simulink library "lego_nxt_lib"  (Simulink 7.5)
settings: Solver=ode45  SolverMode=SingleTasking  StartTime=0.0  StopTime=10.0  RelTol=1e-3
undefined symbols (not defined in the file or in its folder): Copy_of_lego_nxt_lib, PWM
libraries: simulink x1
settings Model: Creator=cmcart01  LastModifiedBy=jpeytonj

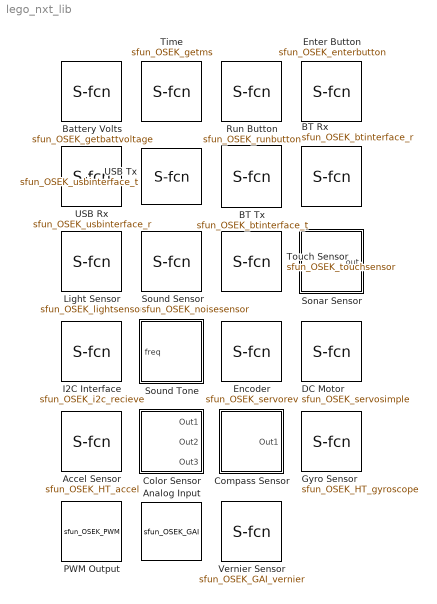
== system lego_nxt_lib ==
  Accel Sensor : S-Function  FunctionName=sfun_OSEK_HT_accel  Parameters=port, st  EnableBusSupport=off  mask(HiTechnic Acceleration Sensor){port=Port 1, st=-1}
      mask prompts: st "Sample time (-1 for inherited):"
      mask help: Outputs acceleration data in three axes (x, y and z) [uint16] representing forward, lateral and vertical directions respectively. The outputs are given in the range 0 to 1023 with a scale factor of ~200 units per g.
      mask init:
      | port_disp(gcb)
      mask Help:
      | The <b>Acceleration Sensor</b> block is an interface for the HiTechnic
      | Accelerometer for the Lego NXT brick.  This sensor can detect values in
      | three axes: x (or pitch), y (or roll) and z.  Pitch represents the angle
      | above or below the horizontal, while roll represents the angle left or
      | right of perfectly vertical.  The z-axis represents lean forward or
      | backward.
      mask StyleString: popup(Port 1|Port 2|Port 3|Port 4),edit
      mask Display:
      | image(imread('ht.jpg'))
      | port_label('output', 1, 'x')
      | port_label('output', 2, 'y')
      | port_label('output', 3, 'z')
      | text(0.1,0.15,'1')
  Analog Input : S-Function  FunctionName=sfun_OSEK_GAI  Parameters=port,gain,intercept,sign,st  EnableBusSupport=off  mask(Generic Analog Input for Mindstorms){port=Port 3, units=Raw ADC count [uint16]; range [0 1023], gain=1, intercept=0, sign=0, st=-1}
      mask prompts: units "Units of Measure:"; sign "Signed output"; st "Sample time (-1 for inherited)"
      mask help:
      | y = ((ADC count)*Gain + Intercept) / 100000.
      | The linear gain and intercept calibration constants are automatically defined for any specified sensor, but may be entered manually for the 'User Defined' measurement option.
      mask init:
      | port_disp(gcb)
      | sens_disp(gcb)
      mask Help:
      | The <b>Generic Analog Input</b> block is an interface for most of the
      | Mindstorms sensors for the Lego NXT brick.
      | 
      | The calibrated output, y, uses linear scaling according to: y = ((ADC count)*Gain + Intercept) / 100000
      | 
      | The relevant values are set automatically according to Mindstorms' documentation which may be found <a href="http://lejos-osek.sourceforge.net/ecrobot_c_api_frame.htm">here</a>
      mask StyleString: popup(Port 1|Port 2|Port 3|Port 4),popup(User defined|Raw ADC count [uint16]; range [0 1023]|Voltage [int16]; range [0 5]V|Light Intensity [uint16]; range [0 1023]|Sound Intensity [uint16]; range [0 1023]),edit,edit,edit,edit
      mask CallbackString:
      | |set_param(gcb,'MaskEnables',{'on','on','off','off','off','on'});
      | temp = get_param(gcb, 'MaskValues');
      | switch get_param(gcb,'units')
      | %NOTE: These are in no particular order as of now
      |     case 'Raw ADC count [uint16]; range [0 1023]'
      |         temp{3} = '1';
      |         temp{4} = '0';
      |         temp{5} = '0';
      |     case 'Voltage [int16]; range [0 5]V'
      |         temp{3} = '.00489';
      |         temp{4} = '0';
      |         temp{5} = '1';
      |     case 'Light Intensity [uint16]; range [0 1023]'
      |         temp{3} = '-1';
      |         temp{4} = '1023';
      |         temp{5} = '0';
      |     case 'Sound Intensity [uint16]; range [0 1023]'
      |         temp{3} = '-1';
      |         temp{4} = '1023';
      |         temp{5} = '0';
      |     case 'User Defined'
      |         set_param(gcb,'MaskEnables',{'on','on','on','on','off','on'});
      |     otherwise
      |         temp{3} = '1';
      |         temp{4} = '0';
      |         temp{5} = '0';
      | end;
      | 
      | set_param(gcb, 'MaskValues', temp);||||
      mask Display:
      | text(0.1,0.15,'3');
      | disp('Raw ADC Count');
  BT Rx : S-Function  AncestorBlock=lego_nxt_lib/USB Rx  FunctionName=sfun_OSEK_btinterface_r  Parameters=init_y0, st  EnableBusSupport=off  mask(Bluetooth Rx Interface    ){init_y0=zeros(32,1,'uint8'), mos=Slave, ip=0, st=-1}
      mask prompts: init_y0 "Initial Output [32x1]uint8:"; mos "Master or Slave"; ip "Slave Device Address:"; st "Sample Time (-1 for inherited):"
      mask help: Receives uint8 vector data via Bluetooth connection. The 'size' secondary output returns the number of bytes received in the last transmission [uint8]. Do not send more than 32 bytes in one timestep; doing so may cause unexpected functionality.
      mask Help:
      | The <b>BT Rx Interface</b> block allows the Lego NXT brick to easily recieve
      | data from an outside machine via Bluetooth. This block should be used only once
      | in a model. It can only receive byte vectors (uint8 vectors). The size
      | output gives the size of the vector received from the current connection.
      | Max vector size for recieve is 32 bytes
      mask StyleString: edit,popup(Master|Slave),edit,edit
      mask CallbackString:
      | |switch (get_param(gcb,'mos'))
      |     case 'Slave'
      |     set_param(gcb,'MaskEnables',{'on','on','off','on'});
      |     set_param(gcb,'MaskVisibilities',{'on','on','off','on'});
      |     case 'Master'
      |     set_param(gcb,'MaskEnables',{'on','on','on','on'});
      |     set_param(gcb,'MaskVisibilities',{'on','on','on','on'});
      | end
      | 
      | ||
      mask Display:
      | image(imread('bt.jpg'), [.2,.1,.6,.8])
      | port_label('output', 1, 'Rx')
      | port_label('output', 2, 'size')
  BT Tx : S-Function  FunctionName=sfun_OSEK_btinterface_t  EnableBusSupport=off  mask(Bluetooth Tx Interface){mos=Slave, ip=0}
      mask prompts: mos "Master or Slave:"; ip "Slave Device Address:"
      mask help: Transmits uint8 vector data via Bluetooth connection. Do not send more than 64 bytes in one timestep; doing so may cause unexpected functionality.
      mask Help:
      | The <b>BT Tx Interface</b> block allows the Lego NXT brick to easily transmit
      | data to an outside machine via Bluetooth. This block should be used only once
      | in a model. It can only transmit byte vectors (uint8 vectors). Max vector
      | size for transmit is 32 bytes.
      mask StyleString: popup(Master|Slave),edit
      mask CallbackString:
      | switch (get_param(gcb,'mos'))
      |     case 'Slave'
      |     set_param(gcb,'MaskEnables',{'on','off'});
      |     set_param(gcb,'MaskVisibilities',{'on','off'});
      |     case 'Master'
      |     set_param(gcb,'MaskEnables',{'on','on'});
      |     set_param(gcb,'MaskVisibilities',{'on','on'});
      | end
      | |
      mask Display:
      | image(imread('bt.jpg'), [.2,.1,.6,.8])
      | port_label('input', 1, 'Tx')
  Battery Volts : S-Function  FunctionName=sfun_OSEK_getbattvoltage  Parameters=st  EnableBusSupport=off  mask(Battery Voltage){st=-1}
      mask prompts: st "Sample time (-1 for inherited):"
      mask help: Outputs current source voltage of battery in mV [uint16].
      mask Help:
      | The <b>Battery Voltage</b> block will output the current source voltage at
      | the battery in mV.  For example, an output of 9000 represents 9.0 V.
      | Maximum value is ideally 9000.
      mask Display: image(imread('volt.jpg'),[.2,.2,.6,.6],'on')
  Color Sensor : Subsystem  mask(HiTechnic Color Sensor V2){port=Port 1, st=-1}
      mask prompts: st "Sample time (-1 for inherited)"
      mask help: Outputs red, green, and blue color saturation values [int16]. Values of each element range from 0-255.
      mask init:
      | port_disp(gcb)
      mask Help:
      | The <b>Color Sensor </b> block reads raw data from a color sensor and
      | extracts the RGB value of a color from that data. The values of each hue are
      | ranged between 0 and 255, as per normal RGB format. This block does not
      | implement the "color number" format supported by the color sensor.
      mask StyleString: popup(Port 1|Port 2|Port 3|Port 4),edit
      mask Display:
      | image(imread('htc.jpg'))
      | text(0.1,0.15,'1')
      | port_label('output', 1, 'r')
      | port_label('output', 2, 'g')
      | port_label('output', 3, 'b')
  Compass Sensor : Subsystem  mask(HiTechnic Compass Sensor   ){port=Port 1, st=-1}
      mask prompts: st "Sample time (-1 for inherited):"
      mask help: Outputs directional data [S16] relative to the closest magnetic source (or magnetic north, by default) in the range of [1,179].
      mask init:
      | port_disp(gcb)
      mask Help:
      | The <b>Compass Sensor</b> block is an interface for HiTechnic's Compass
      | for the Lego NXT brick.  This sensor determines the direction your robot is
      | pointing, which is referred to as the compass heading. The compass outputs
      | a range of values from 1-179, which equals the compass heading divided
      | by 2. The compass may be subject to interference from other magnetic
      | devices, including the brick and motors of the robot itself, so it is
      | important to mount the sensor at least 6 inches away from these objects.
      mask StyleString: popup(Port 1|Port 2|Port 3|Port 4),edit
      mask Display:
      | image(imread('ht.jpg'))
      | text(0.1,0.15,'1')
  DC Motor : S-Function  FunctionName=sfun_OSEK_servosimple  Parameters=port,brake  EnableBusSupport=off  mask(Servo Motor (Simple)){port=Port A, brake=Coast}
      mask prompts: brake "When power=0..."
      mask help: Sets the applied motor voltage [int8] as a percentage (in the range -100..100) of battery voltage. Applying a negative voltage will cause the motor to turn in the reverse direction. Note that motor speed depends not only on applied voltage, but also on motor load.
      mask init:
      | port_disp(gcb)
      mask Help:
      | The <b>DC Motor</b> block is a simplified interface for setting
      | Servo Motor speed.
      mask StyleString: popup(Port A|Port B|Port C),popup(Coast|Brake)
      mask Display:
      | image(imread('servo.jpg'))
      | text(0.1,0.15,'A')
  Encoder : S-Function  FunctionName=sfun_OSEK_servorev  Parameters=port, st  EnableBusSupport=off  mask(Encoder){port=Port A, st=-1}
      mask prompts: st "Sample time (-1 for inherited):"
      mask help: Counts encoder pulses and outputs the motor rotation angle [int32] in degrees relative to the motor's angular position when the model was started.
      mask init:
      | port_disp(gcb)
      mask Help:
      | The <b>Encoder</b> block is a simplified interface for getting the
      | revolution count of a Lego NXT Servo Motor.
      mask StyleString: popup(Port A|Port B|Port C),edit
      mask Display:
      | image(imread('servo.jpg'))
      | text(0.1,0.15,'A')
  Enter Button : S-Function  FunctionName=sfun_OSEK_enterbutton  Parameters=st  EnableBusSupport=off  mask(Enter Button){st=-1}
      mask prompts: st "Sample time (-1 for inherited):"
      mask help: Outputs 1 if enter button is pressed, else 0 [uint8].
      mask Help:
      | The <b>Enter Button</b> block is an interface for the Lego NXT brick's
      | 'Enter' button, or orange button.  This block will output a 1 when the
      | orange button is pressed, and a 0 when the button is unpressed.
      mask Display: image(imread('enter.jpg'))
  Gyro Sensor : S-Function  FunctionName=sfun_OSEK_HT_gyroscope  Parameters=port, st  EnableBusSupport=off  mask(HiTechnic Gyroscopic Sensor){port=Port 1, st=-1}
      mask prompts: st "Sample time (-1 for inherited):"
      mask help: Outputs raw A/D gyroscope data [uint16] in the vertical direction in the range of 0..1023 (offset of ~615). Output is equal to offset plus or minus rotation in degrees/second.
      mask init:
      | port_disp(gcb)
      mask Help:
      | The <b>Gyroscopic Sensor</b> block is an interface for HiTechnic's Gyroscope
      | for the Lego NXT brick.  This sensor detects change in angle at a rate of
      | up to plus or minus 360 degrees per second, and can be read up to 300 times
      | per second.  This sensor operates with an offset of ~615, meaning that the
      | sensor will output a value of 615 when at complete rest.  Its output values
      | range from 0 to 1023.
      mask StyleString: popup(Port 1|Port 2|Port 3|Port 4),edit
      mask Display:
      | image(imread('ht.jpg'))
      | text(0.1,0.15,'1')
  "I2C Interface " : S-Function  FunctionName=sfun_OSEK_i2c_recieve  Parameters=port,addr,intreg,buflen,st  EnableBusSupport=off  mask(I2C Bus Interface (Rx)){port=Port 1, addr=1, intreg=68, buflen=2, st=-1}
      mask prompts: addr "Address:"; intreg "Internal Register (in decimal):"; buflen "Buffer Length:"; st "Sample Time (-1 for inherited)"
      mask help: Outputs data [uint8] read from a slave device of the I2C. Content and width of the output depend on the type of device. This block only supports reading; for writing, use the Tx block.
      mask init:
      | port_disp(gcb)
      mask Help:
      | The <b>I2C Bus Interface (Rx) </b> block facilitates the reception of data from
      | devices linked to the Lego NXT brick through the I2C. Based on the device
      | it is linked to, it creates and outputs a data buffer with information read
      | from the device.  It is recommened that this block be used in tandem with a
      | MATLAB Embedded Fucntion or any other block that can process the data buffer
      mask StyleString: popup(Port 1|Port 2|Port 3|Port 4),edit,edit,edit,edit
      mask Display:
      | image(imread('iic.jpg'))
      | text(0.1,0.15,'1')
      | port_label('output',1,'Rx')
  Light Sensor : S-Function  FunctionName=sfun_OSEK_lightsensor  Parameters=port, st  EnableBusSupport=off  mask(Light Sensor){port=Port 1, st=-1}
      mask prompts: st "Sample time (-1 for inherited):"
      mask help: Outputs a measure of the sensed light on a scale of 0 (dark) to 1023 (bright) [uint16].
      mask init:
      | port_disp(gcb)
      mask Help:
      | The <b>Light Sensor</b> block is an interface for the Lego NXT brick's
      | Light Sensor.  This block gives raw A/D output directly from the sensor,
      | after inverting the data.  In this block, 1023 is the value which
      | represents the brightest or most reflective surface, while a 0 represents
      | the darkest or dullest surface.
      mask StyleString: popup(Port 1|Port 2|Port 3|Port 4),edit
      mask Display:
      | image(imread('light.jpg'))
      | text(0.1,0.15,'1')
  PWM Output : S-Function  AncestorBlock=Copy_of_lego_nxt_lib/PWM  FunctionName=sfun_OSEK_PWM  Parameters=port,reverse  EnableBusSupport=off  mask(PWM Output){port=Port A, reverse=off}
      mask prompts: reverse "Reverse Polarity"
      mask help: Sets the applied PWM duty cycle [uint8] in the range [0..100]. The PWM amplitude is defined by the battery voltage. The PWM signal appears between pins 1 and 2 of the specified output port. The voltage polarity is reversed if the 'reverse polarity' checkbox is selected.
      mask init:
      | port_disp(gcb)
      mask Help: The <b>PWM Output</b> block is a masked version of the DC Motor block
      mask StyleString: popup(Port A|Port B|Port C),checkbox
      mask Display:
      | text(0.35,0.5,'PWM')
      | text(0.1,0.15,'A')
  Run Button : S-Function  FunctionName=sfun_OSEK_runbutton  Parameters=st  EnableBusSupport=off  mask(Run Button){st=-1}
      mask prompts: st "Sample time (-1 for inherited):"
      mask help: Outputs 1 if run button is pressed, else 0 [uint8].
      mask Help:
      | The <b>Run Button<b> block is an interface for the Lego NXT brick's 'run'
      | button, or the gray button to the right of the center orange button.  This
      | block will output a 1 if this button is pressed, and a 0 if this button is
      | unpressed.
      mask Display: image(imread('run.jpg'))
  Sonar Sensor : Subsystem  mask(Sonar Sensor){port=Port 1, statussrc=Hide, st=-1}
      mask prompts: statussrc "Ready Status Output:"; st "Sample time (-1 for inherited):"
      mask help: Outputs the distance (in range 0..255cm) [int16] to the closest object in view. If sensor is not ready, the output distance is set to -1 and the optional 'ready' status output port [boolean] is set to 0.
      mask init:
      | status_cb(gcb,statussrc)
      | port_disp(gcb)
      mask Help:
      | The <b>Sonar Sensor</b> block is an interface for the Lego NXT brick's
      | Ultrasonic Sensor.  It outputs a value between -1 and 255, which represents
      | the distance to the closest sensed object in centimeters (or -1 if the
      | sensor is not ready to output).  The sensor also has a 'ready flag' output,
      | which will output 1 if the sensor is ready, and 0 if it is not ready.
      mask StyleString: popup(Port 1|Port 2|Port 3|Port 4),popup(Show|Hide),edit
      mask CallbackString:
      | |switch get_param(gcb,'statussrc')
      |     case 'Show'
      |         set_param(gcb,'MaskDisplay',sprintf('image(imread(''sonar.jpg''))\ntext(0.1,0.15,''1'')\nport_label(''output'',2,''size'')'));
      |     case 'Hide'
      |         set_param(gcb,'MaskDisplay',sprintf('image(imread(''sonar.jpg''))\ntext(0.1,0.15,''1'')'));
      | end|
      mask Display:
      | image(imread('sonar.jpg'))
      | text(0.1,0.15,'1')
  Sound Sensor : S-Function  FunctionName=sfun_OSEK_noisesensor  Parameters=port, st  EnableBusSupport=off  mask(Sound Sensor){port=Port 1, st=-1}
      mask prompts: st "Sample time (-1 for inherited):"
      mask help: Outputs a measure of the sensed sound on a scale of 0 (quiet) to 1023 (loud) [uint16].
      mask init:
      | port_disp(gcb)
      mask Help:
      | The <b>Sound Sensor</b> block is an interface for the Lego NXT brick's
      | Sound Sensor.  Outputs range from 0 to 1023, where 1023 is the loudest
      | possible sound and 0 is complete silence.
      mask StyleString: popup(Port 1|Port 2|Port 3|Port 4),edit
      mask Display:
      | image(imread('sound.jpg'))
      | text(0.1,0.15,'1')
  Sound Tone : Subsystem  mask(Sound Tone){freqsrc=External, freq=0, volsrc=Internal, vol=70}
      mask prompts: freqsrc "Frequency Source:"; freq "Frequency (in range 31..2100 Hz):"; volsrc "Volume Source:"; vol "Volume (in range 0..100):"
      mask help: Sounds a tone from the Lego NXT brick. The frequency [uint32] and volume [uint8] can be defined either internally as fixed parameter values, or externally as time-varying input signals.
      mask init:
      | voltone_cb(gcb,volsrc,vol,freqsrc,freq);
      mask Help:
      | The <b>Sound Tone</b> block is a flexible interface for the Lego NXT
      | brick's onboard speaker. Each argument (frequency and volume) can be
      | sent to the block as an input or a parameter. The frequency input should be
      | a value between 31 and 2100 (these are audible). The final argument, volume, is a
      | value between 0 and 100.
      mask StyleString: popup(External|Internal),edit,popup(External|Internal),edit
      mask CallbackString:
      | en = get_param(gcb,'MaskEnables');
      | vis = get_param(gcb,'MaskVisibilities');
      | switch get_param(gcb,'freqsrc')
      |   case 'External'
      |     en{2} = 'off';
      |     vis{2} = 'off';
      |   case 'Internal'
      |     en{2} = 'on';
      |     vis{2} = 'on';
      | end
      | set_param(gcb,'MaskEnables',en)
      | set_param(gcb,'MaskVisibilities',vis)||en = get_param(gcb,'MaskEnables');
      | vis = get_param(gcb,'MaskVisibilities');
      | switch get_param(gcb,'volsrc')
      |   case 'External'
      |     en{4} = 'off';
      |     vis{4} = 'off';
      |   case 'Internal'
      |     en{4} = 'on';
      |     vis{4} = 'on';
      | end
      | set_param(gcb,'MaskEnables',en)
      | set_param(gcb,'MaskVisibilities',vis)|
      mask Display:
      | image(imread('tone.jpg'));
      | port_label('input',1,'freq')
  Time : S-Function  FunctionName=sfun_OSEK_getms  Parameters=st  EnableBusSupport=off  mask(System Clock){st=-1}
      mask prompts: st "Sample time (-1 for inherited):"
      mask help: Outputs time in ms since model was started [uint32].
      mask Help:
      | The <b>System Clock</b> block is an interface for the Lego NXT brick's
      | built-in system clock.  This block outputs the 'systick', or the number of
      | milliseconds that have passed since the operating system was loaded.  This
      | clock can be reset upon entry into the program by setting its initial
      | condition.  By default, this clock <u>WILL NOT</u> start at 0 upon entry
      | into the program.
      mask Display: image(imread('clock.jpg'),[.1,.1,.8,.8],'on')
  Touch Sensor : S-Function  FunctionName=sfun_OSEK_touchsensor  Parameters=port, st  EnableBusSupport=off  mask(Touch Sensor){port=Port 1, st=-1}
      mask prompts: st "Sample time (-1 for inherited):"
      mask help: Outputs 1 if pressed, else 0 [uint8].
      mask init:
      | port_disp(gcb)
      mask Help:
      | The <b>Touch Sensor</b> block is an interface for the Lego NXT brick's
      | Touch Sensor button.  When this button is depressed, this block will output
      | a 1, otherwise it will output a 0.
      mask StyleString: popup(Port 1|Port 2|Port 3|Port 4),edit
      mask Display:
      | image(imread('touch.jpg'))
      | text(0.1,0.15,'1')
  USB Rx : S-Function  FunctionName=sfun_OSEK_usbinterface_r  Parameters=init_y0, st  EnableBusSupport=off  mask(USB Rx Interface    ){init_y0=zeros(64,1,'uint8'), st=-1}
      mask prompts: init_y0 "Initial Output [64x1]uint8:"; st "Sample Time (-1 for inherited):"
      mask help: Receives uint8 vector data via USB connection. The 'size' secondary output returns the number of bytes received in the last transmission [uint8]. Do not send more than 64 bytes in one timestep; doing so may cause unexpected functionality.
      mask Help:
      | The <b>USB Rx Interface</b> block allows the Lego NXT brick to easily recieve
      | data from an outside machine via USB. This block should be used only once
      | in a model. It can only receive byte vectors (uint8 vectors). The size
      | output gives the size of the vector received from the current connection.
      | Max vector size for recieve is 64 bytes
      mask Display:
      | image(imread('usb.jpg'))
      | port_label('output', 1, 'Rx')
      | port_label('output', 2, 'size')
  USB Tx : S-Function  AncestorBlock=lego_nxt_lib/USB Tx Interface  FunctionName=sfun_OSEK_usbinterface_t  EnableBusSupport=off
      mask Type: USB Tx Interface
      mask Description: Transmits uint8 vector data via USB connection. Do not send more than 64 bytes in one timestep; doing so may cause unexpected functionality.
      mask Help:
      | The <b>USB Tx Interface</b> block allows the Lego NXT brick to easily transmit
      | data to an outside machine via USB. This block should be used only once in a
      | model. It can only transmit byte vectors (uint8 vectors). Max vector size
      | for transmit is 64 bytes.
      mask Display:
      | image(imread('usb.jpg'))
      | port_label('input', 1, 'Tx')
  Vernier Sensor : S-Function  FunctionName=sfun_OSEK_GAI_vernier  Parameters=port,gain,intercept,sign,st  EnableBusSupport=off  mask(Generic Analog Input for Vernier){port=Port 1, units=Raw ADC count [uint16]; range [0 1023], gain=100000, intercept=0, sign=0, st=-1}
      mask prompts: units "Units of Measure:"; sign "Signed output"; st "Sample time(-1 for inherited):"
      mask help:
      | y = ((ADC count)*Gain + Intercept) / 100000.
      | The linear gain and intercept calibration constants are automatically defined for any specified sensor, but may be entered manually for the 'User Defined' measurement option.
      mask init:
      | port_disp(gcb)
      | vsens_disp(gcb)
      mask Help:
      | The <b>Generic Analog Input</b> block is an interface for most of the
      | Vernier sensors for the Lego NXT brick.
      | 
      | The calibrated output, y, uses linear scaling according to: y = ((ADC count)*Gain + Intercept) / 100000,
      | where the Gain and Intercept values should be entered as 100,000 times their nominal values to avoid floating point computations and to conform to Vernier's calibration protocol.
      | 
      | The relevant values are set automatically according to Vernier's documentation which may be found <a href="http://www.vernier.com/nxt/vernier_sensor_block_2.0.zip">here</a>
      mask StyleString: popup(Port 1|Port 2|Port 3|Port 4),popup(User defined|Raw ADC count [uint16]; range [0 1023]|Voltage [int16]; range [-6 6]V|Current [int16]; range [-.6 .6]A|Acceleration [int16]; range [-50 50] m/s^2|Force [int16]; range [-10 10]N|Light Intensity [uint16]; range [0 600]lx|Temperature [int16]; range [-50 150]C|Pressure [uint16]; range [0 200]kPa|Air Pressure [uint16]; range [80 110]kPa|Wind Speed [unit16]; range [0 30]m/s|pH [uint16]; range [0 14]pH),edit,edit,edit,edit
      mask CallbackString:
      | |set_param(gcb,'MaskEnables',{'on','on','off','off','off','on'});
      | temp = get_param(gcb, 'MaskValues');
      | switch get_param(gcb,'units')
      | %NOTE: These are in no particular order as of now
      |     case 'Raw ADC count [uint16]; range [0 1023]'
      |         temp{3} = '100000';
      |         temp{4} = '0';
      |         temp{5} = '0';
      |     case 'Voltage [int16]; range [-6 6]V'
      |         temp{3} = '-1283';
      |         temp{4} = '695200';
      |         temp{5} = '1';
      |     case 'Force [int16]; range [-10 10]N'
      |         temp{3} = '-2730';
      |         temp{4} = '157000';
      |         temp{5} = '1';
      |     case 'Pressure [uint16]; range [0 200]kPa'
      |         temp{3} = '23820';
      |         temp{4} = '-482800';
      |         temp{5} = '0';
      |     case 'Current [int16]; range [-.6 .6]A'
      |         temp{3} = '-123';
      |         temp{4} = '67870';
      |         temp{5} = '1';
      |     case 'Light Intensity [uint16]; range [0 600]lx'
      |         temp{3} = '74390';
      |         temp{4} = '-1525000';
      |         temp{5} = '0';
      |     case 'Temperature [int16]; range [-50 150]C'
      |         temp{3} = '28930';
      |         temp{4} = '-7118000';
      |         temp{5} = '1';
      |     case 'Wind Speed [unit16]; range [0 30]m/s'
      |         temp{3} = '4000';
      |         temp{4} = '-938800';
      |         temp{5} = '0';
      |     case 'Air Pressure [uint16]; range [80 110]kPa'
      |         temp{3} = '3824';
      |         temp{4} = '8048000';
      |         temp{5} = '0';
      |     case 'Acceleration [int16]; range [-50 50] m/s^2'
      |         temp{3} = '14000';
      |         temp{4} = '-7500000';
      |         temp{5} = '1';
      |     case 'pH [uint16]; range [0 14]pH'
      |         temp{3} = '-1935';
      |         temp{4} = '1423000';
      |         temp{5} = '0';
      |     case 'User defined'
      |         set_param(gcb,'MaskEnables',{'on','on','on','on','off','on'});
      |     otherwise
      |         temp{3} = '100000';
      |         temp{4} = '0';
      |         temp{5} = '1';
      | end;
      | 
      | set_param(gcb, 'MaskValues', temp);||||
      mask Display:
      | text(0.1,0.15,'1');
      | disp('Raw ADC Count');

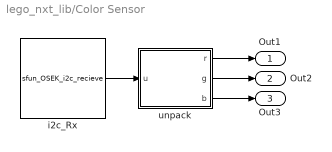
== system lego_nxt_lib/Color Sensor ==
  i2c_Rx : S-Function  FunctionName=sfun_OSEK_i2c_recieve  Parameters=port,1,66,14,st  EnableBusSupport=off
  unpack : Stateflow chart  TreatAsAtomicUnit=on
  Out1 : Outport
  Out2 : Outport  Port=2
  Out3 : Outport  Port=3
  wires:
  unpack/3(b) -> Out3/1
  unpack/2(g) -> Out2/1
  unpack/1(r) -> Out1/1
  i2c_Rx/1 -> unpack/1(u)

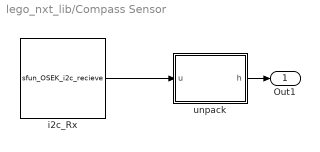
== system lego_nxt_lib/Compass Sensor ==
  i2c_Rx : S-Function  FunctionName=sfun_OSEK_i2c_recieve  Parameters=port,1,65,5,st  EnableBusSupport=off
  unpack : Stateflow chart  TreatAsAtomicUnit=on
  Out1 : Outport
  wires:
  unpack/1(h) -> Out1/1
  i2c_Rx/1 -> unpack/1(u)

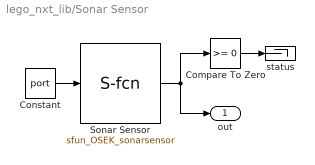
== system lego_nxt_lib/Sonar Sensor ==
  Compare To Zero : simulink/Logic and Bit Operations/Compare To Zero  SystemSampleTime=-1  relop=>=  LogicOutDataTypeMode=boolean
  Constant : Constant  Value=port  SampleTime=st
  Sonar Sensor : S-Function  FunctionName=sfun_OSEK_sonarsensor  Parameters=st  EnableBusSupport=off
  status : Terminator
  out : Outport
  wires:
  Sonar Sensor/1 -> Compare To Zero/1, out/1
  Compare To Zero/1 -> status/1
  Constant/1 -> Sonar Sensor/1

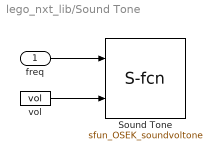
== system lego_nxt_lib/Sound Tone ==
  freq : Inport
  Sound Tone : S-Function  FunctionName=sfun_OSEK_soundvoltone  EnableBusSupport=off
  vol : Constant  Value=vol  OutDataTypeMode=uint8  OutDataTypeStr=uint8
  wires:
  vol/1 -> Sound Tone/2
  freq/1 -> Sound Tone/1

== matlab function Color Sensor/unpack ==
  data: u input double; r output int16 size=1; g output double size=1; b output double size=1
function [r,g,b] = unpack(u)
%#eml

r = typecast(u(3:4),'int16');
g = typecast(u(5:6),'int16');
b = typecast(u(7:8),'int16');

== matlab function Compass Sensor/unpack ==
  data: u input double; h output double size=1
function h = unpack(u)
%#eml

h = typecast(u(4:5),'int16');
